simulink model "sl_groundvehicleDynamics_2025a"  (R2025a)
settings: Solver=ode45  StartTime=0.0  StopTime=2000  RelTol=1e-5  EnableMultiTasking=on
InitFcn:
  | mdl_robot;
values from neighbouring files (symbols this model uses):
  complete_path = complete_path(any(complete_path ~= 0, 2), :)    [startupGround.m]    (also in workspace.mat = [2 3.7 5.2 6.6 7.9 8.9 10.9 12.9 14.9 16.9 18.9 20.9 ... (14)
  obstacles = [26 8 45 5 5 14 35 32 23 45 35 21 ... (36 elements, 12x3)]    [obstacles_air_ground.mat]    (also in workspace.mat)
  optimal_waypoints = [0 -6 -470 -302 -166 215 199 391 404 279 244 0 ... (22 elements, 11x2)]    [matlab.mat]    (also in startupGround.m = [init_state; optimal_waypoints]; startupGround_tester.m = optimize_waypoints(waypoints, init_state); workspace.mat = [2  2; 33  4; 50  20; 43  38; 14  22; 6  38])
  robot =     [matlab.mat]    (also in workspace.mat)
  scan_angles = linspace(-pi/3,pi/3,50)    [startupGround.m]    (also in workspace.mat = [-1.0471975512 -1.004454794 -0.961712036813 -0.918969279622 )
libraries: mobileRoboticsLib x5, simulink x4, simulink_extras x2
settings Model: Creator=sriramn  LastModifiedBy=dinal
settings SolverCC: ZeroCrossAlgorithm=Adaptive  AlgebraicLoopSolver=TrustRegion
settings DataIOCC: LimitDataPoints=on  SaveFormat=Array  ReturnWorkspaceOutputs=off
settings OptimizationCC: ReuseModelBlockBuffer=off  LifeSpan=inf
settings DebuggingCC: SolverPrmCheckMsg=warning  UnconnectedInputMsg=warning  UnconnectedOutputMsg=warning  UnconnectedLineMsg=warning  AllowSymbolicDim=off  SFUnexpectedBacktrackingDiag=warning  SFNoUnconditionalDefaultTransitionDiag=warning  SFExecutionAtInitializationDiag=none  ArithmeticOperatorsInVariantConditions=warning
settings HardwareCC: ProdBitPerPointer=32.0  ProdBitPerSizeT=32.0  ProdBitPerPtrDiffT=32.0  ProdLargestAtomicFloat=None  ProdIntDivRoundTo=Undefined  ProdEndianess=Unspecified  ProdWordSize=32.0  ProdHWDeviceType=32-bit Generic
settings ModelReferenceCC: EnableRefExpFcnMdlSchedulingChecks=on  ModelReferenceMinAlgLoopOccurrences=on  PropagateSignalLabelsOutOfModel=off
settings SFSimCC: SimUseLocalCustomCode=off  CustomCodeUndefinedFunction=UseInterfaceOnly
settings RTWCC: RTWUseLocalCustomCode=off  GPUComputeCapability=3.5
settings CodeAppCC: StateflowObjectComments=on
settings GRTTargetCC: TargetLangStandard=C89/C90 (ANSI)
settings ConfigComp: CovMetricSettings=dw  CovSaveCumulativeToWorkspaceVar=on  CovSaveSingleToWorkspaceVar=on  CovExternalEMLEnable=off  CovSFcnEnable=off
settings SimscapeCC: SimscapeLogDecimation=1  SimscapeNormalizeSystem=off  SimscapeLogDataHistory=5000
settings ConfigurationSet: Description=SimMechanics 2G
settings ExplorerConfigSet: InternalSimMechanicsExplorerSettings="<ExplorerConfiguration><canonicalview>planar_xy</canonicalview><AnimationSetting><BasePlaybackSpeed>1.0</BasePlaybackSpeed><PlaybackSpeedFactor>1.0</PlaybackSpeedFactor></AnimationSetting><TilePanel><TileInfo><Tiles Columns=\"1\" Count=\"1\" Rows=\"1\"><Column Left=\"2\" Weight=\"1\"/><Column Left=\"1628\"/><Row Top=\"2\" Weight=\"1\"/><Row Top=\"1072\"/><Tile Height=\"1\" Width=\"1\" X=\"0\" Y=\"0\"/></Tiles></TileInfo><SceneInfo><SceneViewer><BGColor><R>0.60000002384185791</R><G>0.60000002384185791</G><B>0.60000002384185791</B></BGColor><Camera><Position><X>0.22951840878551699</X><Y>0.32651610611526627</Y><Z>-0.27215421354393321</Z></Position><Center><X>-0.15775714411666431</X><Y>-0.15462825985839526</Y><Z>0.065702552916005602</Z></Center><Up><X>-0.56030137557930915</X><Y>0.72817587161684794</Y><Z>0.39474329445726858</Z></Up><Left>-0.21481383955700509</Left><Right>0.21481383955700509</Right><Bottom>-0.27569784609469139</Bottom><Top>0.27569784609469139</Top></Camera></SceneViewer></SceneInfo></TilePanel></ExplorerConfiguration>"

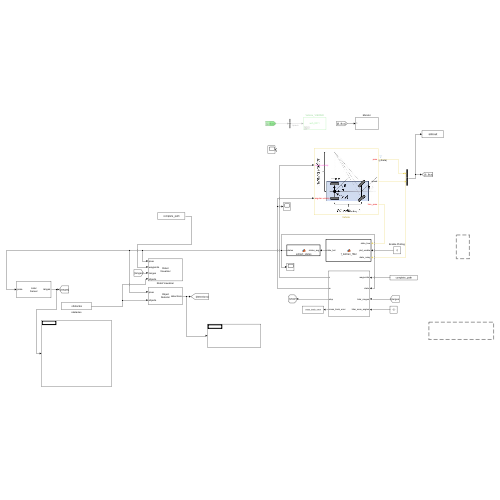
[thumbnail: Simulink's stored preview of the top-level diagram]
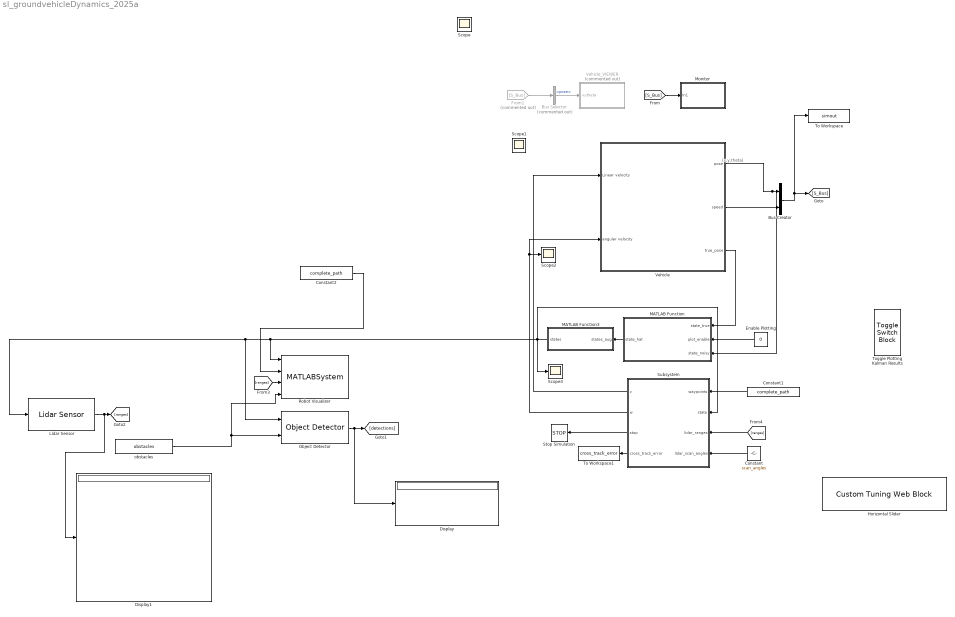
== system sl_groundvehicleDynamics_2025a ==
  note: (x,y,theta)
  Bus Creator : BusCreator  Inputs=2
  Bus Selector : BusSelector  Commented=on  OutputSignals=pose
  Constant : Constant  Value=scan_angles
  Constant1 : Constant  Value=complete_path
  Constant2 : Constant  Value=complete_path
  Display : Display
  Display1 : Display
  Enable Plotting : Constant  Value=0
  From1 : From  Commented=on  GotoTag=S_Bus
  Horizontal Slider : CustomTuningWebBlock  LabelPosition=Hide  ShowInitialText=on  Configuration="{\"components\":[{\"name\":\"LinearScaleComponent\",\"settings\":{\"bounds\":{\"max\":180,\"min\":0,\"tickInterval\":\"auto\"},\"internalTickHeightScaleFactor\":0.5,\"labelColor\":[255,255,200],\"labelFont\":{\"font\":\"Arial\",\"fontSize\":12},\"labelOffset\":0.05,\"labelTransparency\":1,\"needleImage\":{\"size\":[596,842],\"src\":\"data:image\\/svg+xml;base64,PD94bWwgdmVyc2lvbj0iMS4wIiBlbmNvZGluZz0idXRmLTgiPz4NCjwhLS0gR2VuZXJhdG9yOiBBZG9iZSBJbGx1c3RyYXRvciAyNS4wLjAsIFNWRyBFeHBvcnQgUGx1Zy1JbiAuIFNWRyBWZXJzaW9uOiA2LjAwIEJ1aWxkIDApICAtLT4NCjxzdmcgdmVyc2lvbj0iMS4xIg0KCSBpZD0ic3ZnOCIgeG1sbnM6Y2M9Imh0dHA6Ly9jcmVhdGl2ZWNvbW1vbnMub3JnL25zIyIgeG1sbnM6ZGM9Imh0dHA6Ly9wdXJsLm9yZy9kYy9lbGVtZW50cy8xLjEvIiB4bWxuczppbmtzY2FwZT0iaHR0cDovL3d3dy5pbmtzY2FwZS5vcmcvbmFtZXNw ...(+2420 chars)\",\"srcOrientation\":\"Right\"},\"needleOffset\":[-0.8044596912521441,-0.0642123287671233],\"needleSize\":{\"height\":0.4337797619047619,\"width\":0.07668067226890757},\"position\":[0.2829861111111111,0.04398634453781513,0.9196428571428571,0.6088789682539683],\"referencePoint\":\"auto\",\"scaleColors\":[],\"scaleColorsSize\":0.2,\"scaleDirection\":\"LR\",\"showLabels\":1,\"showMinorTicks\":0,\"showSpanLine\":1,\"showTicks\":1,\"tickColor\":[252,252,197],\"tickTransparency\":1,\"valueBarColor\":[0,114,189],\"valueBarOffset\":-0.27,\"valueBarSize\":0.1,\"valueBarTransparency\":1}},{\"name\":\"BackgroundImageComponent\",\"settings\":{\"image\":{\"size\":[380,101],\"src\":\"data:image\\/svg+xml;base64,PHN2ZyB4bWxucz0iaHR0cDovL3d3dy53My5vcmcvMjAwMC9zdmciIHhtbG5zOnhsaW5rPSJodHRwOi8vd3d3LnczLm9yZy8xOTk5L3hsaW5rIiB2aWV3Qm94PSIwIDAgMzgwIDEwMSI+PGRlZnM+PHN0eWxlPi5jbHMtMXtmaWxsOiMwMDJiNDI7fS5jbHMtMntmaWxsOiM0MjcwODI7fS5jbHMtM3tmaWxsOnVybCgjcmFkaWFsLWdyYWRpZW50KTt9LmNscy00e2ZpbGw6I2M4YzhjODtzdHJva2U6IzAwMDt9PC9zdHlsZT48cmFkaWFsR3JhZGllbnQgaWQ9InJhZGlhbC1ncmFkaWVudCIgY3g9IjE5MCIgY3k9IjUwLjUiIHI9IjI2OS4yMSIgZ3JhZGllbnRVbml0cz0idXNlclNwYWNlT25Vc2UiPjxzdG9wIG9mZnNldD0iMC4wMSIgc3RvcC1jb2xvcj0iIzNlNGY1OCIvPjxzdG9wIG9mZnNldD0iMC4wNiIgc3RvcC1jb2xvcj0iIzQ0NTc2MSIvPjxzdG9wIG9mZnNldD0iMC4xNSIgc3RvcC1jb2xvcj0iIzU1NmE3NiIvPjxzdG9wIG9mZnNldD0iMC4yNSIgc3RvcC1jb2xvcj0iIzZkODg5NSIvPjxzdG9wIG9mZnNldD0iMC4zOCIgc3RvcC1jb2xvcj0iIzhmYjJjMyIvPjxzdG9wIG9mZnNldD0iMC41MiIgc3RvcC1jb2xvcj0iI2I2ZTRmYSIvPjxzdG9wIG9mZnNldD0iMSIgc3RvcC1jb2xvcj0iIzE1NDY1NyIvPjwvcmFkaWFsR3JhZGllbnQ+PC9kZWZzPjxnIGlkPSJmcmFtZSI+PGcgaWQ9IkxheWVyXzIiIGRhdGEtbmFtZT0iTGF5ZXIgMiI+PGcgaWQ9IkxheWVyXzEtMiIgZGF0YS1uYW1lPSJMYXllciAxLTIiPjxyZWN0IGlkPSJyZWN0MTAzNiIgY2xhc3M9ImNscy0xIiB4PSIxMSIgeT0iMTEiIHdpZHRoPSIzNTgiIGhlaWdodD0iNzkiLz48cGF0aCBpZD0icGF0aDEwMzgiIGNsYXNzPSJjbHMtMiIgZD0iTTgsOFY5M0gzNzJWOFpNMzY5LDkwSDExVjExSDM2OVoiLz48cGF0aCBpZD0icGF0aDEwNDAiIGNsYXNzPSJjbHMtMyIgZD0iTTAsMFYxMDFIMzgwVjBaTTM3Miw5M0g4VjhIMzcyWiIvPjwvZz48L2c+PC9nPjxnIGlkPSJ0cmFjayI+PHBhdGggaWQ9InJlY3QxNjExIiBjbGFzcz0iY2xzLTQiIGQ9Ik0zMy4zNywyNi41OUgzNDYuNjNjNCwwLDcuMjUsMi42LDcuMjUsNS44MWgwYzAsMy4yMS0zLjI1LDUuODItNy4yNSw1LjgySDMzLjM3Yy00LDAtNy4yNS0yLjYxLTcuMjUtNS44MmgwQzI2LjEyLDI5LjE5LDI5LjM3LDI2LjU5LDMzLjM3LDI2LjU5WiIvPjwvZz48L3N2Zz4=\",\"srcOrientation\":\"horizontal\"},\"position\":[0,0,1,1],\"scaleMode\":\"0\"}},{\"name\":\"ForegroundImageComponent\",\"settings\":{\"image\":{\"size\":[0,0],\"src\":\"default\",\"srcOrientation\":[]},\"isForeground\":1,\"position\":[0,0,1,1],\"scaleMode\":\"0\"}}],\"derived\":{\"blockParameters\":{\"ForegroundColor\":[0.9882352941176471,0.9882352941176471,0.7725490196078432],\"Limits\":{\"Max\":180,\"Min\":0,\"Ticks\":\"auto\"},\"ScaleColors\":[],\"ScaleDirection\":\"Clockwise\",\"ScaleMax\":180,\"ScaleMin\":0,\"TickInterval\":\"auto\",\"fixedAspectRatio\":\"on\"}},\"settings\":{\"BindingType\":\"param\",\"aspectRatio\":3.7777777777777777,\"backgroundColor\":[0,0,0,\"1\"],\"backgroundOffset\":0,\"backgroundOpacity\":1,\"fixedAspectRatio\":\"on\",\"foregroundColor\":[252,252,196],\"orientation\":\"horizontal\",\"showBackgroundColor\":false,\"value\":0,\"version\":\"R2022b\"},\"type\":\"LinearGauge\"}"
  Lidar Sensor : mobileRoboticsLib/Environments/Lidar Sensor  mapName=lidar_map  sensorOffset=[ 0, 0 ]  scanAngles=scan_angles  maxRange=2
      settings: SourceProductName=Mobile Robotics Simulation Toolbox
  MATLAB Function : MATLAB Function  TreatAsAtomicUnit=on
  MATLAB Function3 : MATLAB Function  TreatAsAtomicUnit=on
  Monitor : Subsystem
  Object Detector : mobileRoboticsLib/Environments/Object Detector  mapName=map  sensorOffset=[ 0, 0 ]  sensorAngle=0  fieldOfView=150*pi/180  maxRange=7  maxDetections=5  sampleTime=-1
      settings: SourceProductName=Mobile Robotics Simulation Toolbox
  Robot Visualizer : MATLABSystem  System=Visualizer2D  robotRadius=0.25  mapName=lidar_map  showTrajectory=on  hasWaypoints=on  hasLidar=on  sensorOffset=[ 0, 0 ]  scanAngles=scan_angles  hasObjDetector=on  objDetectorOffset=[ 0, 0 ]  objDetectorAngle=0  objDetectorFOV=pi / 4  objDetectorMaxRange=5  objectColors=[ 1, 0, 0; 0, 1, 0; 0, 0, 1 ]  objectMarkers=s
      mask Type: Visualizer2D
  Scope{,1..3} (4 alike) : Scope
      Scope1 settings: ActiveDisplayYMinimum=-1.25  ActiveDisplayYMaximum=11.25
      Scope2 settings: ActiveDisplayYMinimum=-27.263802233673328  ActiveDisplayYMaximum=24.358424465912226  DataLoggingVariableName=ScopeData2
      Scope3 settings: ActiveDisplayYMinimum=-6.742776009008649  ActiveDisplayYMaximum=48.296023836748965
      Scope settings: ActiveDisplayYMinimum=0.07  ActiveDisplayYMaximum=0.09
  Stop Simulation : Stop
  Subsystem : Subsystem
  To Workspace : ToWorkspace  VariableName=simout  SaveFormat=Timeseries  SampleTime=-1
  To Workspace1 : ToWorkspace  VariableName=cross_track_error  SaveFormat=Timeseries  SampleTime=-1
  Toggle Plotting Kalman Results : ToggleSwitchBlock
  Vehicle : Subsystem
      mask Display: image('vehicle.jpg');
  Vehicle_VIEWER : Subsystem  Commented=on  mask{wp_mat=optimal_waypoints, veh_ID_num=1, veh_init_xytheta=[robot.X robot.Y robot.Theta], Ts=0.5}
      mask prompts: wp_mat "Waypoint matrix for arena [x_col, y_col] (m)"; veh_ID_num "Vehicle ID number"; veh_init_xytheta "Initial pose [x,y,theta]"; Ts "Sample time for updating animation (secs)"
      mask TypeOptions veh_ID_num: 1 | 2 | 3 | 4
      mask DialogControl Control2 Prompt: Animate simulation of Differential Drive Robot (DDR)
      mask Display: fprintf('veh_ID=%d',veh_ID_num);
  obstacles : Constant  Value=obstacles
  wires:
  [S_Bus] -> Monitor/1(In1)
  From1/1 -> Bus Selector/1
  Vehicle/2(speed) -> Bus Creator/2
  Bus Creator/1 -> To Workspace/1, [S_Bus]
  Bus Selector/1 -> Vehicle_VIEWER/1(xytheta)  "<pose>"
  MATLAB Function/1(state_hat) -> MATLAB Function3/1(states_aug)
  Enable Plotting/1 -> MATLAB Function/2(plot_enable)
  obstacles/1 -> Robot Visualizer/4, Object Detector/2
  MATLAB Function3/1(states) -> Subsystem/2(state), Scope3/1, Robot Visualizer/1, Object Detector/1, Lidar Sensor/1
  Vehicle/1(pose) -> MATLAB Function/3(state_noisy), Bus Creator/1
  Object Detector/1 -> Display/1, [detections]
  Lidar Sensor/1 -> Display1/1, [ranges]
  [ranges] -> Robot Visualizer/3
  Subsystem/1(v) -> Vehicle/1(Linear velocity)
  Subsystem/2(w) -> Vehicle/2(angular velocity), Scope2/1
  Constant1/1 -> Subsystem/1(waypoints)
  Subsystem/3(stop) -> Stop Simulation/1
  Constant2/1 -> Robot Visualizer/2
  [ranges] -> Subsystem/3(lidar_ranges)
  Constant/1 -> Subsystem/4(lidar_scan_angles)
  Vehicle/3(true_pose) -> MATLAB Function/1(state_true)
  Subsystem/4(cross_track_error) -> To Workspace1/1

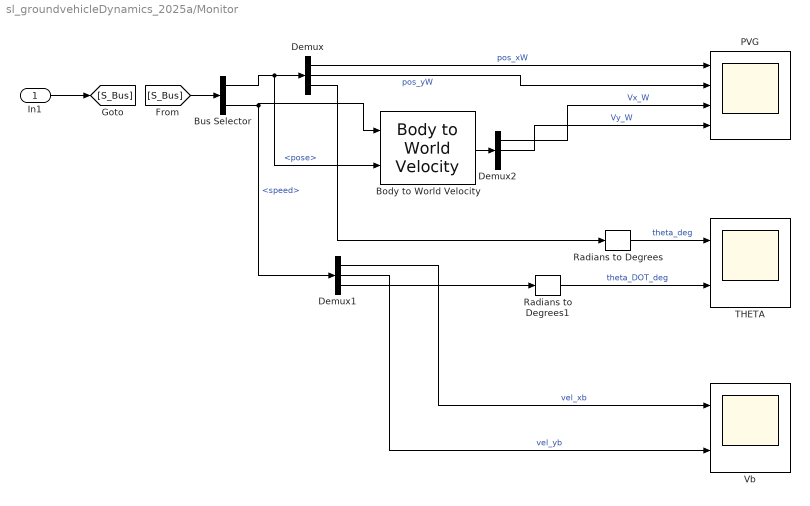
== system sl_groundvehicleDynamics_2025a/Monitor ==
  In1 : Inport
  Body to World Velocity : mobileRoboticsLib/Utilities/Body to World Velocity
      settings: SourceProductName=Mobile Robotics Simulation Toolbox
  Bus Selector : BusSelector  OutputSignals=pose,speed
  Demux : Demux  Outputs=3
  Demux1 : Demux  Outputs=3
  Demux2 : Demux  Outputs=3
  PVG : Scope  NumInputPorts=4
      settings: ActiveDisplayYMinimum=-3.0236  ActiveDisplayYMaximum=27.3548
  Radians to Degrees : simulink_extras/Transformations/Radians to Degrees
  Radians to Degrees1 : simulink_extras/Transformations/Radians to Degrees
  THETA : Scope  NumInputPorts=2
      settings: ActiveDisplayYMinimum=-8.7294  ActiveDisplayYMaximum=60.0661  DataLoggingVariableName=ScopeData2
  Vb : Scope  NumInputPorts=2
      settings: ActiveDisplayYMinimum=0.05577  ActiveDisplayYMaximum=0.8929
  wires:
  In1/1 -> [S_Bus]
  [S_Bus] -> Bus Selector/1
  Demux/1 -> PVG/1  "pos_xW"
  Demux/2 -> PVG/2  "pos_yW"
  Radians to Degrees1/1 -> THETA/2  "theta_DOT_deg"
  Radians to Degrees/1 -> THETA/1  "theta_deg"
  Demux1/3 -> Radians to Degrees1/1
  Demux/3 -> Radians to Degrees/1
  Bus Selector/1 -> Body to World Velocity/2, Demux/1  "<pose>"
  Bus Selector/2 -> Demux1/1, Body to World Velocity/1  "<speed>"
  Body to World Velocity/1 -> Demux2/1
  Demux2/1 -> PVG/3  "Vx_W"
  Demux2/2 -> PVG/4  "Vy_W"
  Demux1/1 -> Vb/1  "vel_xb"
  Demux1/2 -> Vb/2  "vel_yb"

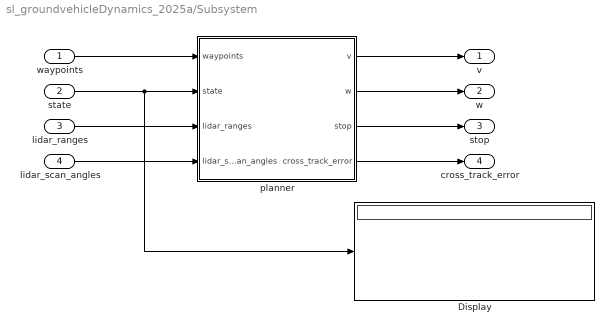
== system sl_groundvehicleDynamics_2025a/Subsystem ==
  waypoints : Inport
  state : Inport  Port=2
  lidar_ranges : Inport  Port=3
  lidar_scan_angles : Inport  Port=4
  Display : Display
  planner : MATLAB Function  TreatAsAtomicUnit=on
  v : Outport
  w : Outport  Port=2
  stop : Outport  Port=3
  cross_track_error : Outport  Port=4
  wires:
  planner/2(w) -> w/1
  planner/1(v) -> v/1
  planner/3(stop) -> stop/1
  waypoints/1 -> planner/1(waypoints)
  state/1 -> Display/1, planner/2(state)
  lidar_ranges/1 -> planner/3(lidar_ranges)
  lidar_scan_angles/1 -> planner/4(lidar_scan_angles)
  planner/4(cross_track_error) -> cross_track_error/1

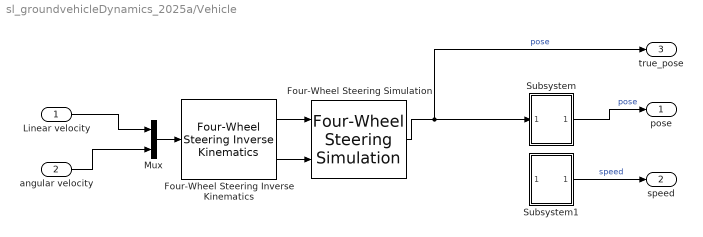
== system sl_groundvehicleDynamics_2025a/Vehicle ==
  Linear velocity : Inport
  angular velocity : Inport  Port=2
  Four-Wheel Steering Inverse Kinematics : mobileRoboticsLib/Kinematic Models/Four-Wheel Steering/Four-Wheel Steering Inverse Kinematics  wheelRadius=0.1  frontWheelDist=0.25  rearWheelDist=0.25  ikMode=Front Steering
      settings: SourceProductName=Mobile Robotics Simulation Toolbox
  Four-Wheel Steering Simulation : mobileRoboticsLib/Kinematic Models/Four-Wheel Steering/Four-Wheel Steering Simulation  wheelRadius=0.1  frontWheelDist=0.25  rearWheelDist=0.25  initX=robot.X  initY=robot.Y  initAngle=robot.Theta  Ts=0.05
      settings: SourceProductName=Mobile Robotics Simulation Toolbox
  Mux : Mux  Inputs=2
  Subsystem : Subsystem
  Subsystem1 : Subsystem
  pose : Outport  VectorParamsAs1DForOutWhenUnconnected=off
  speed : Outport  Port=2
  true_pose : Outport  Port=3  VectorParamsAs1DForOutWhenUnconnected=off
  wires:
  angular velocity/1 -> Mux/2
  Linear velocity/1 -> Mux/1
  Mux/1 -> Four-Wheel Steering Inverse Kinematics/1
  ? -> Subsystem1/1(In1)  "speed"
  Four-Wheel Steering Inverse Kinematics/1 -> Four-Wheel Steering Simulation/1
  Four-Wheel Steering Inverse Kinematics/2 -> Four-Wheel Steering Simulation/2
  Subsystem1/1(speed) -> speed/1  "speed"
  Four-Wheel Steering Simulation/1 -> true_pose/1, Subsystem/1(In1)  "pose"
  Subsystem/1(pose) -> pose/1  "pose"

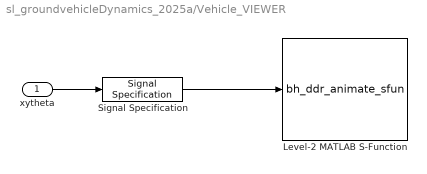
== system sl_groundvehicleDynamics_2025a/Vehicle_VIEWER ==
  xytheta : Inport
  Level-2 MATLAB S-Function : M-S-Function  FunctionName=bh_ddr_animate_sfun  Parameters=Ts, wp_mat, veh_ID_num, veh_init_xytheta
  Signal Specification : SignalSpecification  Dimensions=3
  wires:
  xytheta/1 -> Signal Specification/1
  Signal Specification/1 -> Level-2 MATLAB S-Function/1

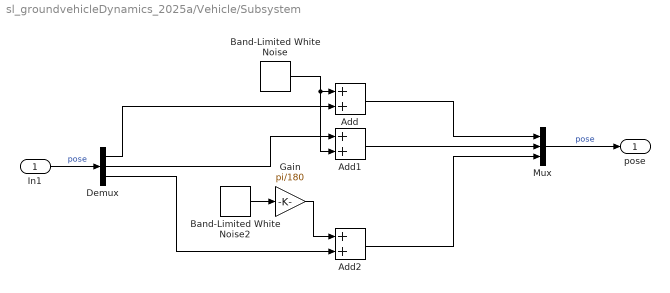
== system sl_groundvehicleDynamics_2025a/Vehicle/Subsystem ==
  In1 : Inport
  Add : Sum
  Add1 : Sum
  Add2 : Sum
  Band-Limited White Noise : simulink/Sources/Band-Limited White Noise  Cov=[0.001]  Ts=0.1  seed=[23341]
  Band-Limited White Noise2 : simulink/Sources/Band-Limited White Noise  Cov=[0.41]  Ts=0.1  seed=[23341]
  Demux : Demux  Outputs=3
  Gain : Gain  Gain=pi/180
  Mux : Mux  Inputs=3
  pose : Outport
  wires:
  Add1/1 -> Mux/2
  Add2/1 -> Mux/3
  Demux/2 -> Add1/1
  Band-Limited White Noise2/1 -> Gain/1
  Demux/3 -> Add2/2
  Band-Limited White Noise/1 -> Add1/2, Add/1
  In1/1 -> Demux/1  "pose"
  Demux/1 -> Add/2
  Gain/1 -> Add2/1
  Mux/1 -> pose/1  "pose"
  Add/1 -> Mux/1

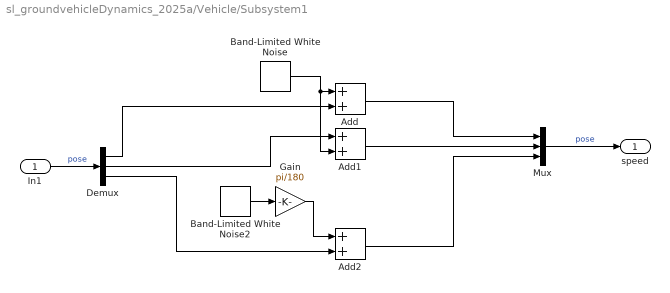
== system sl_groundvehicleDynamics_2025a/Vehicle/Subsystem1 ==
  In1 : Inport
  Add : Sum
  Add1 : Sum
  Add2 : Sum
  Band-Limited White Noise : simulink/Sources/Band-Limited White Noise  Cov=[0.001]  Ts=0.1  seed=[23341]
  Band-Limited White Noise2 : simulink/Sources/Band-Limited White Noise  Cov=[0.41]  Ts=0.1  seed=[23341]
  Demux : Demux  Outputs=3
  Gain : Gain  Gain=pi/180
  Mux : Mux  Inputs=3
  speed : Outport
  wires:
  Add1/1 -> Mux/2
  Add2/1 -> Mux/3
  Demux/2 -> Add1/1
  Band-Limited White Noise2/1 -> Gain/1
  Demux/3 -> Add2/2
  Band-Limited White Noise/1 -> Add1/2, Add/1
  In1/1 -> Demux/1  "pose"
  Demux/1 -> Add/2
  Gain/1 -> Add2/1
  Mux/1 -> speed/1  "pose"
  Add/1 -> Mux/1

== matlab function sl_groundvehicleDynamics_2025a/MATLAB Function ==
  data: state_true input; plot_enable input; state_noisy input; state_hat output
function state_hat  = f_kalman_filter(state_true, plot_enable, state_noisy)
    % [state_hat, k_gain] = kalman_filter(state_noisy);
    state_hat = state_true;
    % persistent idx initialised x_plot y_plot theta_plot error_plot k_plot fig_error fig_analysis max_plot state_true_plot
    % if isempty(initialised)
    %     initialised = 0;
    %     max_plot = 1000;
    %     idx = 0;
    %     x_plot = zeros(1, max_plot);
    %     y_plot = zeros(1, max_plot);
    %     theta_plot = zeros(1, max_plot);
    %     error_plot = zeros(6, max_plot);        
    %     state_true_plot = zeros(6, max_plot);
    %     k_plot = zeros(1, max_plot);
    % 
    % end
    % if plot_enable == 1
    %     fig_error = figure();
    %     fig_analysis = figure();
    %     % Extract estimated states
    %     x_est = state_hat(1);
    %     y_est = state_hat(2);
    %     theta_est = state_hat(6);
    % 
    %     % Circular buffer index
    %     idx = idx + 1;
    %     idx_curr = mod(idx-1, max_plot) + 1;
    % 
    %     % Store data
    %     x_plot(:, idx_curr) = x_est;
    %     y_plot(:, idx_curr) = y_est;
    %     theta_plot(:, idx_curr) = theta_est;
    %     k_plot(:, idx_curr) = k_gain(1,1);
    %     error_plot(1:3, idx_curr) = state_hat(1:3) - state_true(1:3);
    %     state_true_plot(1:3, idx_curr) = state_true;
    % 
    %     % Determine plotting range
    %     if idx <= max_plot
    %         range = 1:idx;
    %     else
    %         range = 1:max_plot;
    %     end
    % 
    %     % Update plots every N steps
    %     plot_update_interval = 10;
    %     if mod(idx, plot_update_interval) == 0 || idx <= 10
    %         %% Figure 1: Estimation, Measurement, Trajectory, Gain
    %         figure(fig_analysis);
    % 
    %         % X position
    %         subplot(2,2,1);
    %         cla;
    %         plot(range, x_plot(1,range), 'b--', 'LineWidth', 2); hold on;
    %         plot(range, state_true_plot(1,range), 'g--', 'LineWidth', 1);
    %         ylabel('x Position');
    %         xlabel('Step');
    %         title('State Estimation - X Position');
    %         legend('Estimated','True','Location','best');
    %         grid on;
    % 
    %         % Y position
    %         subplot(2,2,2);
    %         cla;
    %         plot(range, y_plot(1,range), 'b--', 'LineWidth', 2); hold on;
    %         plot(range, state_true_plot(2,range), 'g--', 'LineWidth', 1);
    %         ylabel('y Position');
    %         xlabel('Step');
    %         title('State Estimation - Y Position');
    %         legend('Estimated','True','Location','best');
    %         grid on;
    % 
    %         % XY trajectory
    %         subplot(2,2,3);
    %         cla;
    %         plot(x_plot(1,range), y_plot(1,range), 'b--', 'LineWidth', 2); hold on;
    %         plot(state_true_plot(1,range), state_true_plot(2,range), 'g--', 'LineWidth', 1);
    %         ylabel('y');
    %         xlabel('x');
    %         title('Trajectory');
    %         legend('Estimated','True','Location','best');
    %         axis equal; grid on;
    % 
    %         % Kalman gain
    %         subplot(2,2,4);
    %         cla;
    %         plot(range, k_plot(1,range), 'r-', 'LineWidth', 2);
    %         ylabel('K(1,1)');
    %         xlabel('Step');
    %         title('Kalman Gain Evolution');
    %         grid on;
    % 
    %         %% Figure 2: Error plots
    %         figure(fig_error);
    % 
    %         % X error
    %         subplot(3,1,1);
    %         cla;
    %         plot(range, error_plot(1,range), 'b-', 'LineWidth', 1.5);
    %         ylabel('x error');
    %         xlabel('Step');
    %         title('Estimation Error - X');
    %         grid on;
    % 
    %         % Y error
    %         subplot(3,1,2);
    %         cla;
    %         plot(range, error_plot(2,range), 'r-', 'LineWidth', 1.5);
    %         ylabel('y error');
    %         xlabel('Step');
    %         title('Estimation Error - Y');
    %         grid on;
    % 
    %         % Theta error
    %         subplot(3,1,3);
    %         cla;
    %         plot(range, error_plot(3,range), 'g-', 'LineWidth', 1.5);
    %         ylabel('\theta error');
    %         xlabel('Step');
    %         title('Estimation Error - Theta');
    %         grid on;
    % 
    %         drawnow;
    %     end
    % end
end

== matlab function sl_groundvehicleDynamics_2025a/Subsystem/planner ==
  data: waypoints input; v output; w output; state input; stop output; lidar_ranges input; lidar_scan_angles input; cross_track_error output
function [v, w, stop, cross_track_error] = f_rvwp(waypoints, state, lidar_ranges, lidar_scan_angles)
    [v, w, stop, cross_track_error] = rvwp(waypoints, state, lidar_ranges, lidar_scan_angles);
end

== matlab function sl_groundvehicleDynamics_2025a/MATLAB Function3 ==
  data: states_aug input; states output
function states = extract_states(states_aug)
    states = states_aug(1:3);
end
